simulink model "TMS_SSORC_2"  (R2022a)
settings: Solver=VariableStepAuto  StartTime=0.0  StopTime=10000  RelTol=1e-3
model workspace: external: MATLAB File parameters_SS.m (data not in the file)
values from neighbouring files (symbols this model uses):
  clnt =     [output_serpentine.mat]    (also in output_straight.mat)
undefined symbols (not defined in the file or in its folder): Con
libraries: fl_lib x27, nesl_utility x9, SimscapeFluids_lib x2, RankineCycle_lib x2, slpidlib x1
settings Model: Creator=victorfernandez  LastModifiedBy=Mick
settings DebuggingCC: UnconnectedInputMsg=warning  UnconnectedOutputMsg=warning  UnconnectedLineMsg=warning
settings RTWCC: DLArmComputeVersion=19.05
settings SimscapeCC: SimscapeLogType=all  SimscapeLogDecimation=2  SimscapeLogLimitData=off

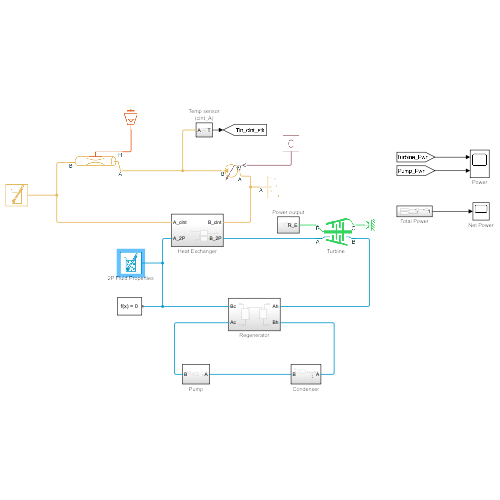
[thumbnail: Simulink's stored preview of the top-level diagram]
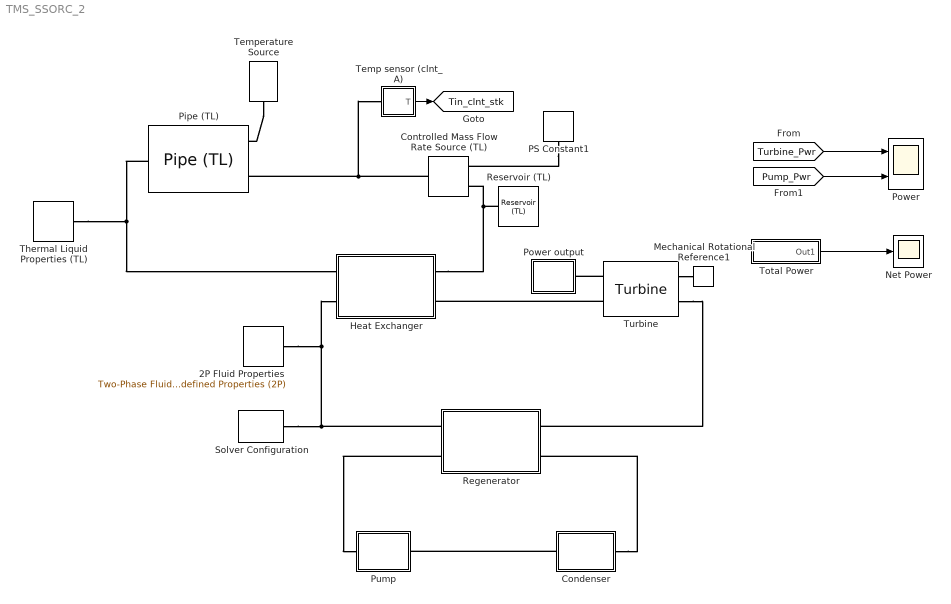
== system TMS_SSORC_2 ==
  2P Fluid Properties : SimscapeFluids_lib/Two-Phase Fluid/Utilities/Two-Phase Fluid Predefined Properties (2P)  fluid=fluids.two_phase_fluid.utilities.enum.Fluid.Isobutane  p_atm=101325 Pa  q_rev=0.01 Pa
      settings: SourceProductBaseCode=SH
  Condenser : Subsystem
  Controlled Mass Flow Rate Source (TL) : fl_lib/Thermal Liquid/Sources/Controlled Mass Flow Rate Source (TL)  area=clch.Ac_tot m^2
      settings: SourceProductBaseCode=PW,SS,VE  InternalSimscapePortConfiguration="{\"Bottom\":[],\"Left\":[{\"id\":\"A\",\"label\":\"A\",\"type\":\"foundation.thermal_liquid.thermal_liquid\"},{\"id\":\"M\",\"label\":\"M\",\"type\":\"input\"}],\"Right\":[{\"id\":\"B\",\"label\":\"B\",\"type\":\"foundation.thermal_liquid.thermal_liquid\"}],\"Top\":[]}"
  Heat Exchanger : Subsystem
  Mechanical Rotational Reference1 : fl_lib/Mechanical/Rotational Elements/Mechanical Rotational Reference
      settings: SourceProductBaseCode=PW,SS,VE
  Net Power : Scope
  PS Constant1 : fl_lib/Physical Signals/Sources/PS Constant  constant=clnt.mdot_tot kg/s
      settings: SourceProductBaseCode=PW,SS,VE
  Pipe (TL) : fl_lib/Thermal Liquid/Elements/Pipe (TL)  length=1 m  area=clch.Ac_tot m^2  Dh=clch.D m  length_add=0.1 m  roughness=15e-6 m  Re_lam=2000  Re_tur=4000  shape_factor=64  Nu_lam=3.66  dynamic_compressibility=simscape.enum.onoff.off  inertia=simscape.enum.onoff.off  p0=0.101325 MPa  T0=293.15 K  mdot0=0 kg/s
      settings: SourceProductBaseCode=PW,SS,VE
  Power : Scope  NumInputPorts=2
  Power output : Subsystem
  Pump : Subsystem
  Regenerator : Subsystem
  Reservoir (TL) : fl_lib/Thermal Liquid/Elements/Reservoir (TL)  pressure_spec=foundation.enum.pressure_spec.atmospheric  reservoir_pressure=0.101325 MPa  reservoir_temperature=293.15 K  area=0.01 m^2
      settings: SourceProductBaseCode=PW,SS,VE
  Solver Configuration : nesl_utility/Solver Configuration  PhysicalDomain=network_engine_domain  SubClassName=solver  LeftPortType=input  RightPortType=generic  Tones=[]  Harmonics=[]  SimulateNoise=off  Profile=off  UseLocalSampling=off  EnableSwitchedLinearOptims=on  FrequencyDomain=off  UseCCode=off  RelTol=0.001  AbsTol=1e-06  MinStep=1e-09  ToWorkspace=off  RevertToSquareIcSolve=off  NumHomotopyIterations=100  PhasorMode=off  PhasorModeNumHarmonics=1  IndexReductionMethod=DerivativeReplacement  DoDC=on  ResidualTolerance=1e-09  UseLocalSolver=off  LocalSolverChoice=NE_BACKWARD_EULER_ADVANCER  LocalSolverSampleTime=0.001  DoFixedCost=off  MaxNonlinIter=3  MaxModeIter=2  ComputeImpulses=off  ImpulseIterations=2  LinearAlgebra=auto  LinearAlgebraNumThread=0  EquationFormulation=NE_TIME_EF  DelaysMemoryBudget=1024  AutomaticFiltering=on  FilteringTimeConstant=0.001  PartitionStorageMethod=AS_NEEDED  PartitionMemoryBudget=1024  PartitionMethod=ROBUST
      settings: SourceProductBaseCode=SS,PW,VE
  Temp sensor (clnt_A) : Subsystem
  Temperature Source : fl_lib/Thermal/Thermal Sources/Temperature Source  temperature=clnt.T_stk_out K
      settings: SourceProductBaseCode=PW,SS,VE
  Thermal Liquid Properties (TL) : SimscapeFluids_lib/Thermal Liquid/Utilities/Thermal Liquid Properties (TL)  fluid_list=fluids.thermal_liquid.utilities.enum.thermal_liquid_fluid_list.water  concentration_param_EG=fluids.thermal_liquid.utilities.enum.thermal_liquid_concentration.volume_fraction  concentration_param_PG=fluids.thermal_liquid.utilities.enum.thermal_liquid_concentration.volume_fraction  c_mass_SW=3.5e-3  c_mass_EG=0.1  c_mass_PG=0.1  c_mass_GL=0.1  c_vol_EG=0.1  c_vol_PG=0.1  beta_const_EG=2.1791 GPa  beta_const_PG=2.1791 GPa  beta_const_GL=2.1791 GPa  p_min_EG=0.01 MPa  p_min_PG=0.01 MPa  p_min_GL=0.01 MPa  p_max_EG=50 MPa  p_max_PG=50 MPa  p_max_GL=50 MPa  p_atm=amb.p Pa
      settings: SourceProductBaseCode=SH
  Total Power : Subsystem
  Turbine : RankineCycle_lib/Turbine  p_A_nominal=1 MPa  p_B_nominal=0.05 MPa  mdot_nominal=ORC.mdot kg/s  v_A_nominal=0.3 m^3/kg  isentropic_efficiency=0.9  mechanical_efficiency=0.9  area_A=Con.PortA_A m^2  area_B=Con.PortA_A * 2 m^2
      settings: SourceProductBaseCode=SS  InternalSimscapePortConfiguration="{\"Bottom\":[],\"Left\":[{\"id\":\"A\",\"label\":\"A\",\"type\":\"foundation.two_phase_fluid.two_phase_fluid\"},{\"id\":\"R\",\"label\":\"R\",\"type\":\"foundation.mechanical.rotational.rotational\"}],\"Right\":[{\"id\":\"B\",\"label\":\"B\",\"type\":\"foundation.two_phase_fluid.two_phase_fluid\"},{\"id\":\"C\",\"label\":\"C\",\"type\":\"foundation.mechanical.rotational.rotational\"}],\"Top\":[]}"
  tag scope: Tin_clnt_stk=global
  wires:
  [Turbine_Pwr] -> Power/1
  [Pump_Pwr] -> Power/2
  Total Power/1(Out1) -> Net Power/1
  Temp sensor (clnt_A)/1(T) -> [Tin_clnt_stk]
  connections:
  Heat Exchanger/RConn1 -- Reservoir (TL)/LConn1 -- Controlled Mass Flow Rate Source (TL)/LConn1
  Thermal Liquid Properties (TL)/RConn1 -- Heat Exchanger/LConn1 -- Pipe (TL)/RConn1
  PS Constant1/RConn1 -- Controlled Mass Flow Rate Source (TL)/LConn2
  Turbine/LConn1 -- Heat Exchanger/RConn2
  Turbine/RConn2 -- Mechanical Rotational Reference1/LConn1
  Turbine/LConn2 -- Power output/LConn1
  Solver Configuration/RConn1 -- 2P Fluid Properties/RConn1 -- Heat Exchanger/LConn2 -- Regenerator/RConn1
  Turbine/RConn1 -- Regenerator/LConn1
  Condenser/LConn1 -- Regenerator/LConn2
  Regenerator/RConn2 -- Pump/RConn1
  Condenser/RConn1 -- Pump/LConn1
  Controlled Mass Flow Rate Source (TL)/RConn1 -- Temp sensor (clnt_A)/LConn1 -- Pipe (TL)/LConn1
  Temperature Source/LConn1 -- Pipe (TL)/LConn2

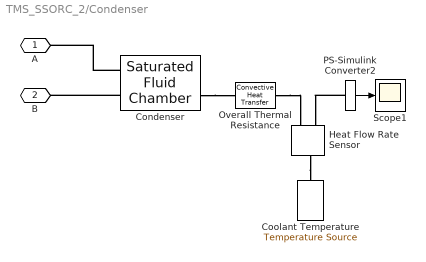
== system TMS_SSORC_2/Condenser ==
  Condenser : RankineCycle_lib/Saturated Fluid Chamber  volume=Con.Fluid_V m^3  area_A=Con.PortA_A m^2  area_B=Con.PortB_A m^2  L_min=0.01  L_max=0.99  p_I_specify=on  p_I_priority=High  p_I=0.02*0 + 0.05 MPa  p_I_nominal_specify=off  p_I_nominal_unit=MPa  p_I_nominal_value=1  L_specify=on  L_priority=High  L=0.8  L_nominal_specify=off  L_nominal_unit=1  L_nominal_value=1
      settings: SourceProductBaseCode=SS  InternalSimscapePortConfiguration="{\"Bottom\":[],\"Left\":[{\"id\":\"A\",\"label\":\"A\",\"type\":\"foundation.two_phase_fluid.two_phase_fluid\"},{\"id\":\"B\",\"label\":\"B\",\"type\":\"foundation.two_phase_fluid.two_phase_fluid\"}],\"Right\":[{\"id\":\"L_out\",\"label\":\"L\",\"type\":\"output\"},{\"id\":\"H\",\"label\":\"H\",\"type\":\"foundation.thermal.thermal\"}],\"Top\":[]}"
  Coolant Temperature : fl_lib/Thermal/Thermal Sources/Temperature Source  temperature=Con.Coolant_T K
      settings: SourceProductBaseCode=PW,SS,VE
  Heat Flow Rate Sensor : fl_lib/Thermal/Thermal Sensors/Heat Flow Rate Sensor
      settings: SourceProductBaseCode=PW,SS,VE
  Overall Thermal Resistance : fl_lib/Thermal/Thermal Elements/Convective Heat Transfer  area=Con.Area m^2  heat_tr_coeff=Con.Heat_Coeff W/(m^2 * K)  T_specify=off  T_priority=None  T=0 K  T_nominal_specify=off  T_nominal_unit=K  T_nominal_value=1  Q_specify=off  Q_priority=None  Q=0 W  Q_nominal_specify=off  Q_nominal_unit=W  Q_nominal_value=1
      settings: SourceProductBaseCode=PW,SS,VE
  PS-Simulink Converter2 : nesl_utility/PS-Simulink Converter  PhysicalDomain=network_engine_domain  SubClassName=ps_output  LeftPortType=input  RightPortType=output  PseudoPeriodic=off  Frequencies=[]  VectorFormat=1-D array  Unit=inherit  AffineConversion=off
      settings: SourceProductBaseCode=SS,PW,VE
  Scope1 : Scope
  A : PMIOPort  Side=Left
  B : PMIOPort  Port=2  Side=Right
  wires:
  PS-Simulink Converter2/1 -> Scope1/1
  connections:
  Condenser/RConn2 -- Overall Thermal Resistance/RConn1
  Condenser/LConn1 -- A/RConn1
  Condenser/LConn2 -- B/RConn1
  Heat Flow Rate Sensor/LConn1 -- Coolant Temperature/LConn1
  PS-Simulink Converter2/LConn1 -- Heat Flow Rate Sensor/RConn1
  Overall Thermal Resistance/LConn1 -- Heat Flow Rate Sensor/RConn2

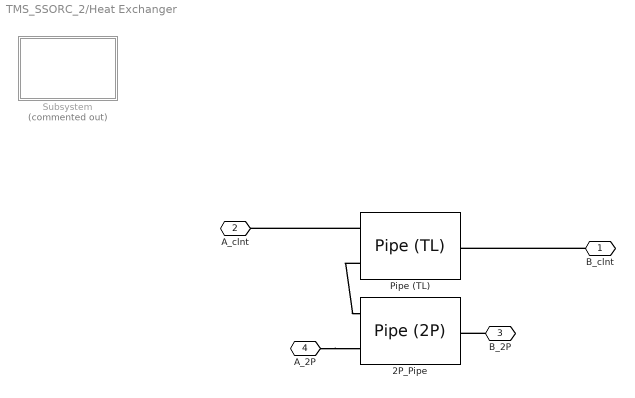
== system TMS_SSORC_2/Heat Exchanger ==
  2P_Pipe : fl_lib/Two-Phase Fluid/Elements/Pipe (2P)  length=10 m  area=Con.PortA_A m^2  Dh=Con.D m  length_add=0.1 m  roughness=15e-6 m  Re_lam=2000  Re_tur=4000  shape_factor=64  Nu_lam=3.66  inertia=simscape.enum.onoff.off  energy_spec=foundation.enum.energy_spec.temperature  p_init=amb.p Pa  T_init=amb.T K  x_init=0.5  alpha_init=0.5  h_init=1500 kJ/kg  u_init=1500 kJ/kg  mdot_init=0 kg/s  time_constant=0.1 s
      settings: SourceProductBaseCode=PW,SS,VE  InternalSimscapePortConfiguration="{\"Bottom\":[],\"Left\":[{\"id\":\"A\",\"label\":\"A\",\"type\":\"foundation.two_phase_fluid.two_phase_fluid\"},{\"id\":\"H\",\"label\":\"H\",\"type\":\"foundation.thermal.thermal\"}],\"Right\":[{\"id\":\"B\",\"label\":\"B\",\"type\":\"foundation.two_phase_fluid.two_phase_fluid\"}],\"Top\":[]}"
  Pipe (TL) : fl_lib/Thermal Liquid/Elements/Pipe (TL)  length=2 m  area=clch.Ac_tot m^2  Dh=clch.D m  length_add=0.1 m  roughness=15e-6 m  Re_lam=2000  Re_tur=4000  shape_factor=64  Nu_lam=4.36  dynamic_compressibility=simscape.enum.onoff.on  inertia=simscape.enum.onoff.off  p0=0.101325 MPa  T0=293.15 K  mdot0=0 kg/s
      settings: SourceProductBaseCode=PW,SS,VE
  Subsystem : Subsystem  Commented=on
  B_clnt : PMIOPort  Side=Right
  A_clnt : PMIOPort  Port=2  Side=Left
  B_2P : PMIOPort  Port=3  Side=Right
  A_2P : PMIOPort  Port=4  Side=Left
  connections:
  Pipe (TL)/LConn2 -- 2P_Pipe/LConn2
  B_clnt/RConn1 -- Pipe (TL)/RConn1
  Pipe (TL)/LConn1 -- A_clnt/RConn1
  B_2P/RConn1 -- 2P_Pipe/RConn1
  A_2P/RConn1 -- 2P_Pipe/LConn1

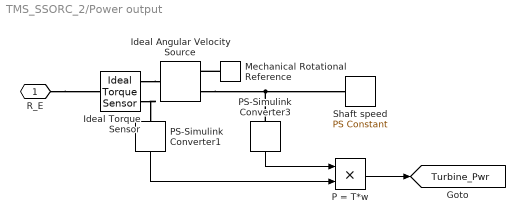
== system TMS_SSORC_2/Power output ==
  Ideal Angular Velocity Source : fl_lib/Mechanical/Mechanical Sources/Ideal Angular Velocity Source
      settings: SourceProductBaseCode=PW,SS,VE
  Ideal Torque Sensor : fl_lib/Mechanical/Mechanical Sensors/Ideal Torque Sensor
      settings: SourceProductBaseCode=PW,SS,VE
  Mechanical Rotational Reference : fl_lib/Mechanical/Rotational Elements/Mechanical Rotational Reference
      settings: SourceProductBaseCode=PW,SS,VE
  P = T*w : Product
  PS-Simulink Converter1 : nesl_utility/PS-Simulink Converter  PhysicalDomain=network_engine_domain  SubClassName=ps_output  LeftPortType=input  RightPortType=output  PseudoPeriodic=off  Frequencies=[]  VectorFormat=1-D array  Unit=N*m  AffineConversion=off
      settings: SourceProductBaseCode=SS,PW,VE
  PS-Simulink Converter3 : nesl_utility/PS-Simulink Converter  PhysicalDomain=network_engine_domain  SubClassName=ps_output  LeftPortType=input  RightPortType=output  PseudoPeriodic=off  Frequencies=[]  VectorFormat=1-D array  Unit=rad/s  AffineConversion=off
      settings: SourceProductBaseCode=SS,PW,VE
  Shaft speed : fl_lib/Physical Signals/Sources/PS Constant  constant=Shaft.speed rpm
      settings: SourceProductBaseCode=PW,SS,VE
  R_E : PMIOPort  Side=Left
  tag scope: Turbine_Pwr=global
  wires:
  PS-Simulink Converter1/1 -> P = T*w/2
  P = T*w/1 -> [Turbine_Pwr]
  PS-Simulink Converter3/1 -> P = T*w/1
  connections:
  Ideal Angular Velocity Source/RConn1 -- PS-Simulink Converter3/LConn1 -- Shaft speed/RConn1
  Ideal Torque Sensor/RConn2 -- PS-Simulink Converter1/LConn1
  R_E/RConn1 -- Ideal Torque Sensor/LConn1
  Mechanical Rotational Reference/LConn1 -- Ideal Angular Velocity Source/RConn2
  Ideal Torque Sensor/RConn1 -- Ideal Angular Velocity Source/LConn1

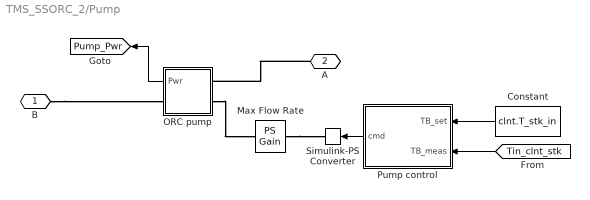
== system TMS_SSORC_2/Pump ==
  Constant : Constant  Value=clnt.T_stk_in
  Max Flow Rate : fl_lib/Physical Signals/Functions/PS Gain  gain=20 kg/s
      settings: SourceProductBaseCode=PW,SS,VE
  ORC pump : Subsystem  mask{power_spec=None, area_A=Con.PortA_A, area_A_unit=m^2, area_B=Con.PortA_A, area_B_unit=m^2, pump_eff=0.9}
      mask prompts: power_spec "Power added"; area_A "Cross-sectional area at port A"; area_B "Cross-sectional area at port B"; pump_eff "Efficiency"
      mask TypeOptions power_spec: Isentropic | None
      mask TypeOptions area_A_unit: m^2 | cm^2 | mm^2
      mask TypeOptions area_B_unit: m^2 | cm^2 | mm^2
  Pump control : Subsystem
  Simulink-PS Converter : nesl_utility/Simulink-PS Converter  PhysicalDomain=network_engine_domain  SubClassName=ps_input  LeftPortType=input  RightPortType=output  PseudoPeriodic=off  Frequencies=[]  NoiseDistribution=none  NoiseParameters=[]  Unit=1  AffineConversion=off  FilteringAndDerivatives=provide  SimscapeFilterOrder=1  InputFilterTimeConstant=0.001  UdotUserProvided=0
      settings: SourceProductBaseCode=SS,PW,VE
  B : PMIOPort  Side=Right
  A : PMIOPort  Port=2  Side=Left
  tag scope: Pump_Pwr=global
  wires:
  ORC pump/1(Pwr) -> [Pump_Pwr]
  Pump control/1(cmd) -> Simulink-PS Converter/1
  Constant/1 -> Pump control/1(TB_set)
  [Tin_clnt_stk] -> Pump control/2(TB_meas)
  connections:
  B/RConn1 -- ORC pump/RConn1
  A/RConn1 -- ORC pump/LConn1
  Max Flow Rate/LConn1 -- Simulink-PS Converter/RConn1
  ORC pump/LConn2 -- Max Flow Rate/RConn1

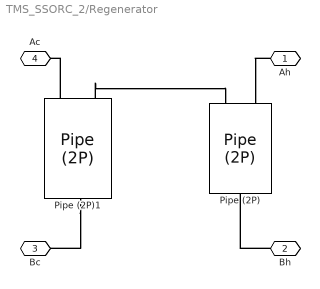
== system TMS_SSORC_2/Regenerator ==
  Pipe (2P) : fl_lib/Two-Phase Fluid/Elements/Pipe (2P)  length=2 m  area=Con.PortA_A m^2  Dh=Con.D m  length_add=0.1 m  roughness=15e-6 m  Re_lam=2000  Re_tur=4000  shape_factor=64  Nu_lam=3.66  inertia=simscape.enum.onoff.off  energy_spec=foundation.enum.energy_spec.temperature  p_init=amb.p Pa  T_init=amb.T K  x_init=0.5  alpha_init=0.5  h_init=1500 kJ/kg  u_init=1500 kJ/kg  mdot_init=0 kg/s  time_constant=0.1 s
      settings: SourceProductBaseCode=PW,SS,VE  InternalSimscapePortConfiguration="{\"Bottom\":[],\"Left\":[{\"id\":\"A\",\"label\":\"A\",\"type\":\"foundation.two_phase_fluid.two_phase_fluid\"},{\"id\":\"H\",\"label\":\"H\",\"type\":\"foundation.thermal.thermal\"}],\"Right\":[{\"id\":\"B\",\"label\":\"B\",\"type\":\"foundation.two_phase_fluid.two_phase_fluid\"}],\"Top\":[]}"
  Pipe (2P)1 : fl_lib/Two-Phase Fluid/Elements/Pipe (2P)  length=2 m  area=Con.PortA_A m^2  Dh=Con.D m  length_add=0.1 m  roughness=15e-6 m  Re_lam=2000  Re_tur=4000  shape_factor=64  Nu_lam=3.66  inertia=simscape.enum.onoff.off  energy_spec=foundation.enum.energy_spec.temperature  p_init=amb.p Pa  T_init=amb.T K  x_init=0.5  alpha_init=0.5  h_init=1500 kJ/kg  u_init=1500 kJ/kg  mdot_init=0 kg/s  time_constant=0.1 s
      settings: SourceProductBaseCode=PW,SS,VE  InternalSimscapePortConfiguration="{\"Bottom\":[],\"Left\":[{\"id\":\"A\",\"label\":\"A\",\"type\":\"foundation.two_phase_fluid.two_phase_fluid\"},{\"id\":\"H\",\"label\":\"H\",\"type\":\"foundation.thermal.thermal\"}],\"Right\":[{\"id\":\"B\",\"label\":\"B\",\"type\":\"foundation.two_phase_fluid.two_phase_fluid\"}],\"Top\":[]}"
  Ah : PMIOPort  Side=Left
  Bh : PMIOPort  Port=2  Side=Left
  Bc : PMIOPort  Port=3  Side=Right
  Ac : PMIOPort  Port=4  Side=Right
  connections:
  Pipe (2P)1/RConn1 -- Bc/RConn1
  Pipe (2P)1/LConn2 -- Pipe (2P)/LConn2
  Pipe (2P)1/LConn1 -- Ac/RConn1
  Ah/RConn1 -- Pipe (2P)/LConn1
  Bh/RConn1 -- Pipe (2P)/RConn1

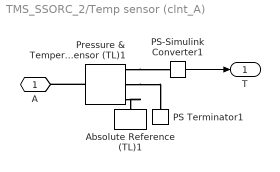
== system TMS_SSORC_2/Temp sensor (clnt_A) ==
  Absolute Reference (TL)1 : fl_lib/Thermal Liquid/Elements/Absolute Reference (TL)
      settings: SourceProductBaseCode=PW,SS,VE
  PS Terminator1 : fl_lib/Physical Signals/Sinks/PS Terminator
      settings: SourceProductBaseCode=PW,SS,VE
  PS-Simulink Converter1 : nesl_utility/PS-Simulink Converter  PhysicalDomain=network_engine_domain  SubClassName=ps_output  LeftPortType=input  RightPortType=output  PseudoPeriodic=off  Frequencies=[]  VectorFormat=1-D array  Unit=K  AffineConversion=off
      settings: SourceProductBaseCode=SS,PW,VE
  Pressure & Temperature Sensor (TL)1 : fl_lib/Thermal Liquid/Sensors/Pressure & Temperature Sensor (TL)
      settings: SourceProductBaseCode=PW,SS,VE  InternalSimscapePortConfiguration="{\"Bottom\":[],\"Left\":[{\"id\":\"A\",\"label\":\"A\",\"type\":\"foundation.thermal_liquid.thermal_liquid\"}],\"Right\":[{\"id\":\"B\",\"label\":\"B\",\"type\":\"foundation.thermal_liquid.thermal_liquid\"},{\"id\":\"P\",\"label\":\"P\",\"type\":\"output\"},{\"id\":\"T\",\"label\":\"T\",\"type\":\"output\"}],\"Top\":[]}"
  A : PMIOPort  Side=Left
  T : Outport
  wires:
  PS-Simulink Converter1/1 -> T/1
  connections:
  Pressure & Temperature Sensor (TL)1/RConn1 -- Absolute Reference (TL)1/LConn1
  Pressure & Temperature Sensor (TL)1/LConn1 -- A/RConn1
  Pressure & Temperature Sensor (TL)1/RConn2 -- PS Terminator1/LConn1
  Pressure & Temperature Sensor (TL)1/RConn3 -- PS-Simulink Converter1/LConn1

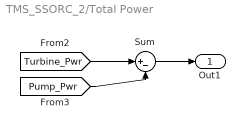
== system TMS_SSORC_2/Total Power ==
  Sum : Sum  Inputs=|+-
  Out1 : Outport
  wires:
  [Turbine_Pwr] -> Sum/1
  [Pump_Pwr] -> Sum/2
  Sum/1 -> Out1/1

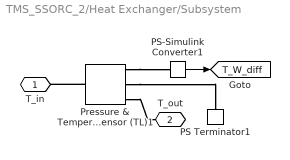
== system TMS_SSORC_2/Heat Exchanger/Subsystem ==
  PS Terminator1 : fl_lib/Physical Signals/Sinks/PS Terminator
      settings: SourceProductBaseCode=PW,SS,VE
  PS-Simulink Converter1 : nesl_utility/PS-Simulink Converter  PhysicalDomain=network_engine_domain  SubClassName=ps_output  LeftPortType=input  RightPortType=output  PseudoPeriodic=off  Frequencies=[]  VectorFormat=1-D array  Unit=K  AffineConversion=off
      settings: SourceProductBaseCode=SS,PW,VE
  Pressure & Temperature Sensor (TL)1 : fl_lib/Thermal Liquid/Sensors/Pressure & Temperature Sensor (TL)
      settings: SourceProductBaseCode=PW,SS,VE  InternalSimscapePortConfiguration="{\"Bottom\":[],\"Left\":[{\"id\":\"A\",\"label\":\"A\",\"type\":\"foundation.thermal_liquid.thermal_liquid\"}],\"Right\":[{\"id\":\"B\",\"label\":\"B\",\"type\":\"foundation.thermal_liquid.thermal_liquid\"},{\"id\":\"P\",\"label\":\"P\",\"type\":\"output\"},{\"id\":\"T\",\"label\":\"T\",\"type\":\"output\"}],\"Top\":[]}"
  T_in : PMIOPort  Side=Left
  T_out : PMIOPort  Port=2  Side=Right
  tag scope: T_W_diff=global
  wires:
  PS-Simulink Converter1/1 -> [T_W_diff]
  connections:
  Pressure & Temperature Sensor (TL)1/RConn2 -- PS Terminator1/LConn1
  Pressure & Temperature Sensor (TL)1/RConn3 -- PS-Simulink Converter1/LConn1
  Pressure & Temperature Sensor (TL)1/RConn1 -- T_out/RConn1
  Pressure & Temperature Sensor (TL)1/LConn1 -- T_in/RConn1

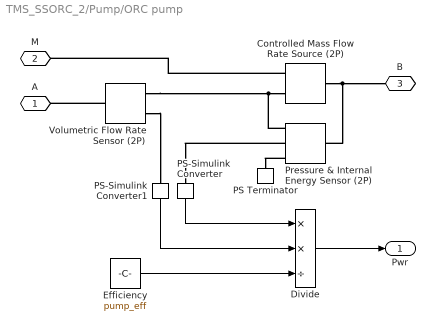
== system TMS_SSORC_2/Pump/ORC pump ==
  Controlled Mass Flow Rate Source (2P) : fl_lib/Two-Phase Fluid/Sources/Controlled Mass Flow Rate Source (2P)  power_spec=foundation.enum.power_spec.isentropic  area_A=0.01 m^2  area_B=0.01 m^2
      settings: SourceProductBaseCode=PW,SS,VE  InternalSimscapePortConfiguration="{\"Bottom\":[],\"Left\":[{\"id\":\"A\",\"label\":\"A\",\"type\":\"foundation.two_phase_fluid.two_phase_fluid\"},{\"id\":\"M\",\"label\":\"M\",\"type\":\"input\"}],\"Right\":[{\"id\":\"B\",\"label\":\"B\",\"type\":\"foundation.two_phase_fluid.two_phase_fluid\"}],\"Top\":[]}"
  Divide : Product  Inputs=**/
  Efficiency : Constant  Value=pump_eff
  PS Terminator : fl_lib/Physical Signals/Sinks/PS Terminator
      settings: SourceProductBaseCode=PW,SS,VE
  PS-Simulink Converter : nesl_utility/PS-Simulink Converter  PhysicalDomain=network_engine_domain  SubClassName=ps_output  LeftPortType=input  RightPortType=output  PseudoPeriodic=off  Frequencies=[]  VectorFormat=inherit  Unit=Pa  AffineConversion=off
      settings: SourceProductBaseCode=SS,PW,VE
  PS-Simulink Converter1 : nesl_utility/PS-Simulink Converter  PhysicalDomain=network_engine_domain  SubClassName=ps_output  LeftPortType=input  RightPortType=output  PseudoPeriodic=off  Frequencies=[]  VectorFormat=inherit  Unit=m^3/s  AffineConversion=off
      settings: SourceProductBaseCode=SS,PW,VE
  Pressure & Internal Energy Sensor (2P) : fl_lib/Two-Phase Fluid/Sensors/Pressure & Internal Energy Sensor (2P)
      settings: SourceProductBaseCode=PW,SS,VE  InternalSimscapePortConfiguration="{\"Bottom\":[],\"Left\":[{\"id\":\"A\",\"label\":\"A\",\"type\":\"foundation.two_phase_fluid.two_phase_fluid\"}],\"Right\":[{\"id\":\"B\",\"label\":\"B\",\"type\":\"foundation.two_phase_fluid.two_phase_fluid\"},{\"id\":\"P\",\"label\":\"P\",\"type\":\"output\"},{\"id\":\"U\",\"label\":\"U\",\"type\":\"output\"}],\"Top\":[]}"
  Volumetric Flow Rate Sensor (2P) : fl_lib/Two-Phase Fluid/Sensors/Volumetric Flow Rate Sensor (2P)
      settings: SourceProductBaseCode=PW,SS,VE  InternalSimscapePortConfiguration="{\"Bottom\":[],\"Left\":[{\"id\":\"A\",\"label\":\"A\",\"type\":\"foundation.two_phase_fluid.two_phase_fluid\"}],\"Right\":[{\"id\":\"B\",\"label\":\"B\",\"type\":\"foundation.two_phase_fluid.two_phase_fluid\"},{\"id\":\"V\",\"label\":\"V\",\"type\":\"output\"}],\"Top\":[]}"
  A : PMIOPort  Side=Left
  M : PMIOPort  Port=2  Side=Left
  B : PMIOPort  Port=3  Side=Right
  Pwr : Outport
  wires:
  Efficiency/1 -> Divide/3
  PS-Simulink Converter1/1 -> Divide/2
  PS-Simulink Converter/1 -> Divide/1
  Divide/1 -> Pwr/1
  connections:
  Pressure & Internal Energy Sensor (2P)/RConn2 -- PS-Simulink Converter/LConn1
  Volumetric Flow Rate Sensor (2P)/RConn2 -- PS-Simulink Converter1/LConn1
  Volumetric Flow Rate Sensor (2P)/LConn1 -- A/RConn1
  Controlled Mass Flow Rate Source (2P)/LConn2 -- M/RConn1
  Pressure & Internal Energy Sensor (2P)/RConn3 -- PS Terminator/LConn1
  Volumetric Flow Rate Sensor (2P)/RConn1 -- Pressure & Internal Energy Sensor (2P)/RConn1 -- Controlled Mass Flow Rate Source (2P)/LConn1
  Controlled Mass Flow Rate Source (2P)/RConn1 -- B/RConn1 -- Pressure & Internal Energy Sensor (2P)/LConn1

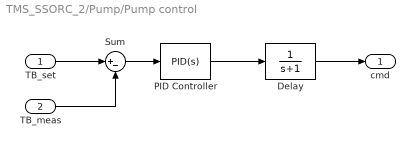
== system TMS_SSORC_2/Pump/Pump control ==
  TB_set : Inport
  TB_meas : Inport  Port=2
  Delay : TransferFcn  Denominator=[1 1]
  PID Controller : slpidlib/PID Controller  Controller=PID  Form=Ideal  TimeDomain=Continuous-time  UseExternalTs=off  SampleTime=-1  IntegratorMethod=Forward Euler  FilterMethod=Forward Euler  ControllerParametersSource=internal  P=-0.244537597157716  I=0.00336610494624602  UseKiTs=off  D=66.0075053065735  N=65.9397633021034  UseFilter=on  TunerSelectOption=Transfer Function Based (PID Tuner App)  InitialConditionSource=internal  InitialConditionForIntegrator=0  InitialConditionForFilter=0  DifferentiatorICPrevScaledInput=0  ExternalReset=none  TrackingMode=off  Kt=1  LimitOutput=on  SatLimitsSource=internal  UpperSaturationLimit=1  LowerSaturationLimit=0  LinearizeAsGain=on  AntiWindupMode=back-calculation  Kb=0.1  POutMin=[]  POutMax=[]  IOutMin=[]  IOutMax=[]  DOutMin=[]  DOutMax=[]  NOutMin=[]  NOutMax=[]  SumOutMin=[]  SumOutMax=[]  SaturationOutMin=[]  SaturationOutMax=[]  PParamMin=[]  PParamMax=[]  IParamMin=[]  IParamMax=[]  DParamMin=[]  DParamMax=[]  NParamMin=[]  NParamMax=[]  KbParamMin=[]  KbParamMax=[]  KtParamMin=[]  KtParamMax=[]  KbOutMin=[]  KbOutMax=[]  KtOutMin=[]  KtOutMax=[]  IntegratorOutMin=[]  IntegratorOutMax=[]  FilterOutMin=[]  FilterOutMax=[]  SumI1OutMin=[]  SumI1OutMax=[]  SumI2OutMin=[]  SumI2OutMax=[]  SumI3OutMin=[]  SumI3OutMax=[]  SumI4OutMin=[]  SumI4OutMax=[]  SumDOutMin=[]  SumDOutMax=[]  DifferentiatorOutMin=[]  DifferentiatorOutMax=[]  FilterDiffOutCoefMin=[]  FilterDiffOutCoefMax=[]  ReciprocalOutMin=[]  ReciprocalOutMax=[]  SumDenOutMin=[]  SumDenOutMax=[]  SumNumOutMin=[]  SumNumOutMax=[]  DivideOutMin=[]  DivideOutMax=[]  UdiffTsProdOutMin=[]  UdiffTsProdOutMax=[]  NTsProdOutMin=[]  NTsProdOutMax=[]  UintegralTsProdOutMin=[]  UintegralTsProdOutMax=[]  UngainTsProdOutMin=[]  UngainTsProdOutMax=[]  IntegratorContinuousStateAttributes=''  IntegratorStateMustResolveToSignalObject=off  IntegratorRTWStateStorageClass=Auto  FilterContinuousStateAttributes=''  FilterStateMustResolveToSignalObject=off  FilterRTWStateStorageClass=Auto  ParallelPVariant=Passthrough  IdealPVariant=InternalParameters  IVariant=InternalParameters  DVariant=InternalParameters  IntegratorVariant=Continuous  SatVariant=Enabled  AWVariant=BackCalculation  PCopyVariant=Disabled  TRVariant=Disabled  FdbkBlocksVariant=Forward  IdealPFdbkVariant=Disabled  SatFdbkVariant=Disabled  DerivativeFilterVariant=ContFilter  NVariant=InternalParameters  NCopyVariant=Disabled  FilterICVariant=InternalICsFilter  IntegratorICVariant=InternalICs  ExternalResetVariant=Disabled  TRSumVariant=Passthrough  SumFdbkVariant=Disabled  SumVariant=Sum_PID  TsampFilterVariant=InternalTs  TsampNgainVariant=Passthrough  TsampIntegralVariant=Passthrough  ExternalSaturationOutDataTypeStr=Inherit: Same as second input  aMode=0
  Sum : Sum  Inputs=|+-
  cmd : Outport
  wires:
  TB_meas/1 -> Sum/2
  TB_set/1 -> Sum/1
  Sum/1 -> PID Controller/1
  Delay/1 -> cmd/1
  PID Controller/1 -> Delay/1
